simulink model "Tim1PWM_Tim3IC"  (R2015b)
settings: Solver=FixedStepDiscrete  StartTime=0.0  StopTime=10.0  FixedStep=0.5  RelTol=1e-3
libraries: USART_Lib x4, TIMERS_Lib x2, STM32_Config_Lib x1
settings Model: Creator=Gang  LastModifiedBy=reynaudp
settings DataIOCC: SaveFormat=Array
settings OptimizationCC: OptimizeModelRefInitCode=on  LifeSpan=1
settings DebuggingCC: UnderspecifiedInitializationDetection=Classic  MergeDetectMultiDrivingBlocksExec=none  SolverPrmCheckMsg=warning
settings HardwareCC: ProdBitPerPointer=32  ProdLargestAtomicInteger=Integer  ProdWordSize=32  ProdHWDeviceType=STMicroelectronics->STM32 32-bit Cortex-M
settings RTWCC: SystemTargetFile=stm32.tlc  TemplateMakefile=stm32.tmf  Description=stm32 (Embedded Target)  GenerateReport=on  LaunchReport=on
settings CodeAppCC: IgnoreCustomStorageClasses=off  MaxIdLength=64  CustomSymbolStrType=$N$R$M  SimulinkBlockComments=off
settings STFCustomTargetCC: CodeReplacementLibrary=ARM CMSIS SIN COS  ParMdlRefBuildCompliant=on  ConcurrentExecutionCompliant=off  IncludeMdlTerminateFcn=off  GeneratePreprocessorConditionals=Use local settings  CombineOutputUpdateFcns=on  ERTCustomFileBanners=on  SupportContinuousTime=off  SupportNonInlinedSFcns=off  MATLABClassNameForMDSCustomization=Simulink.SoftwareTarget.ERTCustomization  CPPClassGenCompliant=off  GRTInterface=off  SystemTargetFile=stm32.tlc
settings ERTTargetCC: CodeReplacementLibrary=ARM CMSIS SIN COS  CompOptLevelCompliant=off  ConcurrentExecutionCompliant=off  IncludeMdlTerminateFcn=off  ERTFirstTimeCompliant=off  ModelStepFunctionPrototypeControlCompliant=off  CPPClassGenCompliant=off  UseToolchainInfoCompliant=off  ERTSrcFileBannerTemplate=sourceFileTemplate.cgt  ERTHdrFileBannerTemplate=sourceFileTemplate.cgt  ERTDataSrcFileTemplate=sourceFileTemplate.cgt  ERTDataHdrFileTemplate=sourceFileTemplate.cgt  ERTCustomFileTemplate=customRoutineProcess.tlc
settings ConfigComp: CovModelRefEnable=Off  CovSFcnEnable=off

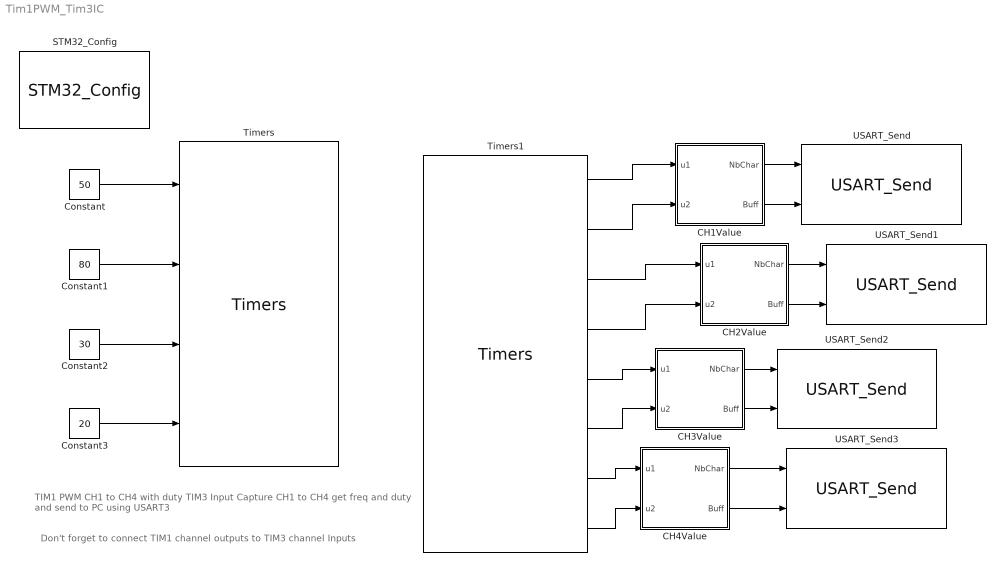
== system Tim1PWM_Tim3IC ==
  note: Don't forget to connect TIM1 channel outputs to TIM3 channel Inputs
  note: TIM1 PWM CH1 to CH4 with duty
      | TIM3 Input Capture CH1 to CH4 get freq and duty and send to PC using USART3
  CH1Value : MATLAB Function  TreatAsAtomicUnit=on
  CH2Value : MATLAB Function  TreatAsAtomicUnit=on
  CH3Value : MATLAB Function  TreatAsAtomicUnit=on
  CH4Value : MATLAB Function  TreatAsAtomicUnit=on
  Constant : Constant  Value=50
  Constant1 : Constant  Value=80
  Constant2 : Constant  Value=30
  Constant3 : Constant  Value=20
  STM32_Config : STM32_Config_Lib/STM32_Config  Priority=0  Project_Path=.\  Config_File=Tim1PWM_Tim3IC.ioc  MCU_Name=STM32F407VGTx
  Timers : TIMERS_Lib/Timers  currentTIM=TIM1  TIM_Name=TIM1  TIM_APBClock=168000000  TIM_CKD=1  TIM_Set_Clk=on  TIM_Prescaler=1  TIM_Clock=42000000.00  Variable_frequency=off  TIM_Set_OutFreq=on  TIM_ARR=2100  Output_frequency=20000.00  Repetition_counter=0  TIM_Mode=Up  TIM_DMA=none  TIM_IRQ=off  TIM_IRQ_ONLY=off  TIM_UP=off  TIM_TRG=off  TIM_COM=off  TIM_BRK=off  NbTIM=2  CH1_enable=on  CH1N_enable=on  CH1_type=Output_PWM  CH1_DMA=off  CH1_int=off  CH1_edge=Rising  CH1_div=1  CH1_variable_duty=on  CH1_set_pulse=off  CH1_output_duty=0.00  CH1_pulse=0  CH2_enable=on  CH2N_enable=on  CH2_type=Output_PWM  CH2_DMA=off  CH2_int=off  CH2_edge=Rising  CH2_div=1  CH2_variable_duty=on  CH2_set_pulse=off  CH2_output_duty=0.00  CH2_pulse=0  CH3_enable=on  CH3N_enable=on  CH3_type=Output_PWM  CH3_DMA=off  CH3_int=off  CH3_edge=Rising  CH3_div=1  CH3_variable_duty=on  CH3_set_pulse=off  CH3_output_duty=0.00  CH3_pulse=0  CH4_enable=on  CH4N_enable=off  CH4_type=Output_PWM  CH4_DMA=off  CH4_int=off  CH4_edge=Rising  CH4_div=1  CH4_variable_duty=on  CH4_set_pulse=off  CH4_output_duty=0.00  CH4_pulse=0
  Timers1 : TIMERS_Lib/Timers  currentTIM=TIM3  TIM_Name=TIM3  TIM_APBClock=84000000  TIM_CKD=1  TIM_Set_Clk=on  TIM_Prescaler=1  TIM_Clock=21000000.00  Variable_frequency=off  TIM_Set_OutFreq=on  TIM_ARR=210000  Output_frequency=100.00  Repetition_counter=0  TIM_Mode=Up  TIM_DMA=none  TIM_IRQ=on  TIM_IRQ_ONLY=off  TIM_UP=off  TIM_TRG=off  TIM_COM=off  TIM_BRK=off  NbTIM=2  CH1_enable=on  CH1N_enable=off  CH1_type=Input_Capture  CH1_DMA=off  CH1_int=on  CH1_edge=Rising_Falling  CH1_div=1  CH1_variable_duty=on  CH1_set_pulse=off  CH1_output_duty=0.00  CH1_pulse=0  CH2_enable=on  CH2N_enable=off  CH2_type=Input_Capture  CH2_DMA=off  CH2_int=on  CH2_edge=Rising_Falling  CH2_div=1  CH2_variable_duty=on  CH2_set_pulse=off  CH2_output_duty=0.00  CH2_pulse=0  CH3_enable=on  CH3N_enable=off  CH3_type=Input_Capture  CH3_DMA=off  CH3_int=on  CH3_edge=Rising_Falling  CH3_div=1  CH3_variable_duty=on  CH3_set_pulse=off  CH3_output_duty=0.00  CH3_pulse=0  CH4_enable=on  CH4N_enable=off  CH4_type=Input_Capture  CH4_DMA=off  CH4_int=on  CH4_edge=Rising_Falling  CH4_div=1  CH4_variable_duty=on  CH4_set_pulse=off  CH4_output_duty=0.00  CH4_pulse=0
  USART_Send{,1..3} (4 alike) : USART_Lib/USART_Send  USART_name=USART3  Buff_size=512  nbUsart=1  usartMode=Asynchronous  usartDma_Rx=off  usartDma_Tx=off  usartIt=on
  wires:
  Constant/1 -> Timers/1
  Constant1/1 -> Timers/2
  Constant2/1 -> Timers/3
  Constant3/1 -> Timers/4
  CH1Value/1(NbChar) -> USART_Send/1
  CH1Value/2(Buff) -> USART_Send/2
  CH2Value/1(NbChar) -> USART_Send1/1
  CH2Value/2(Buff) -> USART_Send1/2
  CH3Value/1(NbChar) -> USART_Send2/1
  CH3Value/2(Buff) -> USART_Send2/2
  CH4Value/1(NbChar) -> USART_Send3/1
  CH4Value/2(Buff) -> USART_Send3/2
  Timers1/1 -> CH1Value/1(u1)
  Timers1/2 -> CH1Value/2(u2)
  Timers1/3 -> CH2Value/1(u1)
  Timers1/4 -> CH2Value/2(u2)
  Timers1/5 -> CH3Value/1(u1)
  Timers1/6 -> CH3Value/2(u2)
  Timers1/7 -> CH4Value/1(u1)
  Timers1/8 -> CH4Value/2(u2)

== matlab function Tim1PWM_Tim3IC/CH2Value ==
  data: u1 input; NbChar output uint16 size=1; Buff output uint32 size=1; u2 input
function [NbChar, Buff] = convert(u1, u2)
if coder.target('Sfun')
% Executing in MATLAB, Buff is null
Buff = uint32(0);
NbChar = uint16(0);
else
% Executing in the generated code. 
CH2Msg = zeros(1,31,'uint8');
coder.ceval('sprintf',coder.wref(CH2Msg),['CH2: %3.3fKHz : %3.3f%%', 13, 10, 0],u1/1000.0,u2);
Buff = coder.ceval('getBuffPtr',coder.wref(CH2Msg));
NbChar = coder.ceval('strlen',coder.ref(CH2Msg));
end
end
%Buff = uint32(y);
%%Buff = [buffer(1:4), tmp, 13, 10, 0];

== matlab function Tim1PWM_Tim3IC/CH1Value ==
  data: u1 input; NbChar output uint16 size=1; Buff output uint32 size=1; u2 input
function [NbChar, Buff] = convert(u1, u2)
if coder.target('Sfun')
% Executing in MATLAB, Buff is null
Buff = uint32(0);
NbChar = uint16(0);
else
% Executing in the generated code. 
%buffer = zeros(1,15,'uint8');
%strLen = int32(0);
%strLen = coder.ceval('sprintf',coder.wref(buffer),['CH1: %3.3f',0],u1/1000.0);
%tmp = uint8('KHz');
%buffer2 = zeros(1,15,'uint8');
%strLen = coder.ceval('sprintf',coder.wref(buffer2),[': %3.3f',0],u2);
%tmp2 = uint8('%');
%CH2Val = [buffer(1:10), tmp, buffer2(1:8), tmp2, 13, 10, 0];
%Buff = uint32(coder.ref(y));
%Buff = coder.ceval('getBuffPtr',coder.ref(CH2Val));
%NbChar = uint16(size(CH2Val,2));


% Executing in the generated code. 
CH1Msg = zeros(1,30,'uint8');
coder.ceval('sprintf',coder.wref(CH1Msg),['CH1: %3.3fKHz : %3.3f%%', 13, 10, 0],u1/1000.0,u2);
Buff = coder.ceval('getBuffPtr',coder.wref(CH1Msg));
NbChar = coder.ceval('strlen',coder.ref(CH1Msg));
end
end
%Buff = uint32(y);
%%Buff = [buffer(1:4), tmp, 13, 10, 0];

== matlab function Tim1PWM_Tim3IC/CH3Value ==
  data: u1 input; NbChar output uint16 size=1; Buff output uint32 size=1; u2 input
function [NbChar, Buff] = convert(u1, u2)
if coder.target('Sfun')
% Executing in MATLAB, Buff is null
Buff = uint32(0);
NbChar = uint16(0);
else
% Executing in the generated code. 
CH3Msg = zeros(1,32,'uint8');
coder.ceval('sprintf',coder.wref(CH3Msg),['CH3: %3.3fKHz : %3.3f%%', 13, 10, 0],u1/1000.0,u2);
Buff = coder.ceval('getBuffPtr',coder.wref(CH3Msg));
NbChar = coder.ceval('strlen',coder.ref(CH3Msg));
end
end
%Buff = uint32(y);
%%Buff = [buffer(1:4), tmp, 13, 10, 0];

== matlab function Tim1PWM_Tim3IC/CH4Value ==
  data: u1 input; NbChar output uint16 size=1; Buff output uint32 size=1; u2 input
function [NbChar, Buff] = convert(u1, u2)
if coder.target('Sfun')
% Executing in MATLAB, Buff is null
Buff = uint32(0);
NbChar = uint16(0);
else
% Executing in the generated code. 
CH4Msg = zeros(1,33,'uint8');
coder.ceval('sprintf',coder.wref(CH4Msg),['CH4: %3.3fKHz : %3.3f%%', 13, 10, 0],u1/1000.0,u2);
Buff = coder.ceval('getBuffPtr',coder.wref(CH4Msg));
NbChar = coder.ceval('strlen',coder.ref(CH4Msg));
end
end
%Buff = uint32(y);
%%Buff = [buffer(1:4), tmp, 13, 10, 0];
